simulink model "cactinhchatphoPRONY"  (Simulink 7.3)
settings: Solver=ode45  StartTime=0.0  StopTime=1  RelTol=1e-3
settings Model: Creator=nthuy  LastModifiedBy=nthuy

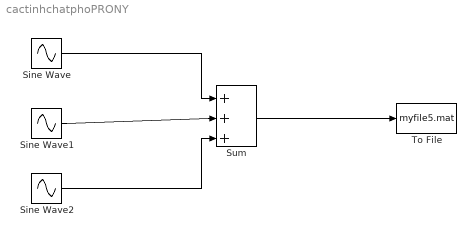
== system cactinhchatphoPRONY ==
  Sine Wave : Sin  Amplitude=2  Bias=0  Frequency=2*pi*100  Phase=pi/6  Samples=10  SampleTime=0  Offset=0
  Sine Wave1 : Sin  Amplitude=1  Bias=0  Frequency=2*pi*150  Phase=0  Samples=10  SampleTime=0  Offset=0
  Sine Wave2 : Sin  Amplitude=1.5  Bias=0  Frequency=2*pi*180  Phase=pi/4  Samples=10  SampleTime=0  Offset=0
  Sum : Sum  Inputs=|+++  OutDataType=fixdt(1, 16)  OutScaling=2^0
  To File : ToFile  Filename=myfile5.mat  MatrixName=xx  SampleTime=0.001
  wires:
  Sine Wave/1 -> Sum/1
  Sine Wave1/1 -> Sum/2
  Sine Wave2/1 -> Sum/3
  Sum/1 -> To File/1
